simulink library "Kitchen_Lib"  (R2023a)
settings: Solver=VariableStepAuto  StartTime=0.0  StopTime=10.0  RelTol=1e-3  EnableMultiTasking=on
undefined symbols (not defined in the file): Kitc_BusTyp_P, Kitc_BusTypSkyr_C, Kitc_ColrLedColrls_C, Kitc_ColrLedGrn_C, Kitc_ColrLedRed_C, Kitc_ColrLedYlw_C, Kitc_StDgnWtrTank_C, Kitc_StElecPlugScktOffByClmp50_P, Kitc_StsDlyBlink_C, Kitc_StsErrBlink_C, Kitc_StsFctAcvn_P, Kitc_StsInfoBlink_C, Kitc_StsKitchnOffAutoIgOff_P, Kitc_StsKitchnOffBySwt_P, Kitc_StsKitchnOffDoorLockd_P, Kitc_StsKitchnOffIgOff_P, Kitc_StsKitchnOffUv_P, Kitc_StsKitchnOnBySwt_P, Kitc_StsKitchnOnNVM_P, Kitc_StsLedOff_C, Kitc_StsLedOn_C, Kitc_StsLrgCnsAcv_P, Kitc_StTrfrAnSwtInstd_P, Kitc_StTrfrSwtInstd_P, Kitc_TiKitcRefgtrOffDly_P, Kitc_ULowrThdBat_C, Kitc_UUpprThdBat_C, Kitc_ValFalse_C, Kitc_ValPwmFreq2_C, Kitc_ValPwmFreq_C, Kitc_ValTrue_C
libraries: MAN_Library x50, E2E_Lib x3
(part 9 of 13)

== system Kitchen_Lib/Kitchen/100ms/Kitchn/Subsystem1/Subsystem19/WaterTankEmptyDiagnostic/TurnOffDelay/TurnOffDelayOriginal ==
  TurnOffDelayEnable : Inport
  TurnOffDelayThreshold : Inport  Port=2
  CycleTime : Inport  Port=3
  Data Type Conversion1 : DataTypeConversion  OutDataTypeStr=uint32  SaturateOnIntegerOverflow=off  RndMeth=Floor
  Data Type Conversion2 : DataTypeConversion  OutDataTypeStr=boolean  SaturateOnIntegerOverflow=off  RndMeth=Floor
  Data Type Conversion3 : DataTypeConversion  OutDataTypeStr=uint32  SaturateOnIntegerOverflow=off  RndMeth=Floor
  FallingEdgeDetection : Subsystem  AncestorBlock=MAN_Library/FallingEdgeDetection
  Logical Operator2 : Logic  Operator=OR  AllPortsSameDT=off  OutDataTypeStr=boolean
  TimePulseOriginal : Subsystem  AncestorBlock=MAN_Library/BasicLibrary/TimePulseOriginal
  TurnOffDelayFlag : Outport
  TurnOffDelayExpiredTime : Outport  Port=2
  wires:
  CycleTime/1 -> TimePulseOriginal/3(CycleTime)
  Data Type Conversion3/1 -> TurnOffDelayExpiredTime/1
  Data Type Conversion1/1 -> TimePulseOriginal/2(TimePulseDuration)
  TurnOffDelayThreshold/1 -> Data Type Conversion1/1
  FallingEdgeDetection/1(Q) -> TimePulseOriginal/1(TimePulseEnable)
  TimePulseOriginal/2(TimePulseExpiredTime) -> Data Type Conversion3/1
  Logical Operator2/1 -> TurnOffDelayFlag/1
  TimePulseOriginal/1(TimePulseFlag) -> Logical Operator2/2
  Data Type Conversion2/1 -> FallingEdgeDetection/1(CLK), Logical Operator2/1
  TurnOffDelayEnable/1 -> Data Type Conversion2/1

== system Kitchen_Lib/Kitchen/100ms/Kitchn/Subsystem1/Subsystem16/001_KitchnCtl/002_FlipFlop/KSW-KitchenControl/KSW_Battery ==
  Kitchn_On : Inport
  "GW_Ubat " : Inport  Port=2
  GW_StClmp15 : Inport  Port=3
  "GW_StUvTopPrio " : Inport  Port=4
  "GW_ModeExbn " : Inport  Port=5
  "GW_StClmp50Off3Sec " : Inport  Port=6
  CLS_StDoorLockdOutd : Inport  Port=7
  Kitc_StsHostsCallAcv : Inport  Port=8
  GW_StEngRung : Inport  Port=9
  ABat_StAddlBatInstd : Inport  Port=10
  BatteryVoltageUnder22.7V : Subsystem
  BatteryVoltageUnder23V : Subsystem
  KitchenActivation : Subsystem
  Logical Operator51 : Logic  Operator=OR  AllPortsSameDT=off  OutDataTypeStr=boolean
  KitchnAcv : Outport
  LrgCnsEna : Outport  Port=2
  LrgCns : Outport  Port=3
  Kitc_WarnLrgCns : Outport  Port=4
  Kitc_StBuzRe : Outport  Port=5
  wires:
  Logical Operator51/1 -> BatteryVoltageUnder23V/2(EngOrAddlBat), KitchenActivation/9(EngOrAddlBat), BatteryVoltageUnder22.7V/2(EngOrAddlBat)
  "GW_Ubat "/1 -> BatteryVoltageUnder23V/1(GW_Ubat), BatteryVoltageUnder22.7V/3("GW_Ubat ")
  BatteryVoltageUnder22.7V/1(BatUUnder22.7V) -> KitchenActivation/5(BatUUnder22.7V)
  BatteryVoltageUnder23V/2(Kitc_WarnLrgCns) -> Kitc_WarnLrgCns/1
  BatteryVoltageUnder23V/3(Kitc_StBuzRe) -> Kitc_StBuzRe/1
  BatteryVoltageUnder23V/1(LrgCnsOff) -> KitchenActivation/6(LrgCnsOff)
  Kitchn_On/1 -> BatteryVoltageUnder22.7V/1(Kitchn_On), [Kitchn_On]
  [Kitchn_On] -> BatteryVoltageUnder23V/3(Kitchn_On)
  Kitc_StsHostsCallAcv/1 -> BatteryVoltageUnder23V/4(Kitc_StsHostsCallAcv)
  "GW_StClmp50Off3Sec "/1 -> KitchenActivation/1("GW_StClmp50Off3Sec ")
  "GW_StUvTopPrio "/1 -> KitchenActivation/2("GW_StUvTopPrio ")
  "GW_ModeExbn "/1 -> KitchenActivation/3("GW_ModeExbn ")
  CLS_StDoorLockdOutd/1 -> KitchenActivation/4(CLS_StDoorLockdOutd)
  GW_StClmp15/1 -> KitchenActivation/8(GW_StClmp15)
  KitchenActivation/1(KitchnAcv) -> KitchnAcv/1
  KitchenActivation/2(LrgCnsEna) -> LrgCnsEna/1
  KitchenActivation/3(LrgCns) -> LrgCns/1
  [Kitchn_On] -> KitchenActivation/7(Kitchn_On)
  ABat_StAddlBatInstd/1 -> Logical Operator51/1
  GW_StEngRung/1 -> Logical Operator51/2

== system Kitchen_Lib/Kitchen/100ms/Kitchn/Subsystem1/Subsystem16/001_KitchnCtl/002_FlipFlop/KSW-KitchenControl/KitchenControl ==
  Kitchn_On : Inport
  KitchnAcv : Inport  Port=2
  LrgCnsEna : Inport  Port=3
  "GW_ModeExbn " : Inport  Port=4
  GW_StClmp15 : Inport  Port=5
  ABat_StAddlBatInstd : Inport  Port=6
  GW_StEngRung : Inport  Port=7
  Constant : Constant  Value=Kitc_BusTypSkyr_C
  Constant1 : Constant  Value=Kitc_BusTypSkyr_C
  Constant2 : Constant  Value=Kitc_BusTyp_P
  Constant3 : Constant  Value=Kitc_BusTyp_P
  Constant4 : Constant  Value=Kitc_ValPwmFreq_C
  Gain : Gain  Gain=100  OutDataTypeStr=uint16
  Gain1 : Gain  Gain=100  OutDataTypeStr=uint16
  Logical Operator5 : Logic  Operator=OR  AllPortsSameDT=off  OutDataTypeStr=boolean
  Logical Operator50 : Logic  Inputs=3  AllPortsSameDT=off  OutDataTypeStr=boolean
  Logical Operator51 : Logic  Operator=OR  AllPortsSameDT=off  OutDataTypeStr=boolean
  Multiport Switch : MultiPortSwitch  DataPortOrder=Zero-based contiguous  Inputs=2  zeroidx=on  SaturateOnIntegerOverflow=off  InputSameDT=off
  Multiport Switch1 : MultiPortSwitch  DataPortOrder=Zero-based contiguous  Inputs=2  zeroidx=on  SaturateOnIntegerOverflow=off  InputSameDT=off
  Relational Operator : RelationalOperator  Operator===  OutDataTypeStr=boolean  InputSameDT=off
  Relational Operator1 : RelationalOperator  Operator===  OutDataTypeStr=boolean  InputSameDT=off
  Kitc_StsKitcAcv : Outport
  Kitchn_HostsCallOn : Outport  Port=2
  Kitc_StLrgCns : Outport  Port=3
  Kitc_StSmlCns : Outport  Port=4
  Kitc_StWtrPump : Outport  Port=5
  Kitc_StKitcLi : Outport  Port=6
  Kitc_StsPwmFreq : Outport  Port=7
  wires:
  Multiport Switch/1 -> Kitchn_HostsCallOn/1, Kitc_StsKitcAcv/1
  GW_StClmp15/1 -> Logical Operator50/1
  Constant/1 -> Relational Operator/2
  Logical Operator50/1 -> [SkylinerKitchnAcv]
  Multiport Switch1/1 -> Gain/1
  "GW_ModeExbn "/1 -> Logical Operator5/1
  Relational Operator1/1 -> Multiport Switch1/1
  Logical Operator5/1 -> Kitc_StKitcLi/1
  KitchnAcv/1 -> Logical Operator5/2, Gain1/1, Kitc_StWtrPump/1, Multiport Switch/2
  Kitchn_On/1 -> Logical Operator50/2
  Constant2/1 -> Relational Operator/1
  Logical Operator51/1 -> Logical Operator50/3
  Constant1/1 -> Relational Operator1/2
  Constant3/1 -> Relational Operator1/1
  Relational Operator/1 -> Multiport Switch/1
  [SkylinerKitchnAcv] -> Multiport Switch1/3
  [SkylinerKitchnAcv] -> Multiport Switch/3
  ABat_StAddlBatInstd/1 -> Logical Operator51/1
  GW_StEngRung/1 -> Logical Operator51/2
  LrgCnsEna/1 -> Multiport Switch1/2
  Gain/1 -> Kitc_StLrgCns/1
  Gain1/1 -> Kitc_StSmlCns/1
  Constant4/1 -> Kitc_StsPwmFreq/1

== system Kitchen_Lib/Kitchen/100ms/Kitchn/Subsystem1/Subsystem16/001_KitchnCtl/002_FlipFlop/KitchenEnable/KitchenOffAutomaticIgnitionOff ==
  Kitc_StDemoBd : Inport
  Kitc_TdOff : Inport  Port=2
  GW_StClmp15 : Inport  Port=3
  Kitchen_On : Inport  Port=4
  "Constant4           " : MAN_Library/TimeConstant  hours=0  minutes=0  seconds=10  miliseconds=0
  Logical Operator36 : Logic  AllPortsSameDT=off  OutDataTypeStr=boolean
  Logical Operator37 : Logic  Operator=NOT  Inputs=4  AllPortsSameDT=off  OutDataTypeStr=boolean
  Multiport Switch2 : MultiPortSwitch  DataPortOrder=Zero-based contiguous  Inputs=2  zeroidx=on  SaturateOnIntegerOverflow=off  InputSameDT=off
  RisingEdgeDetection2 : MAN_Library/RisingEdgeDetection
  Terminator : Terminator
  TurnOnDelay : MAN_Library/TurnOnDelay  CycleTime=Cycle Time: 10 Ms
  "KitchnOffAutoIgOff " : Outport
  wires:
  TurnOnDelay/1 -> RisingEdgeDetection2/1
  RisingEdgeDetection2/1 -> "KitchnOffAutoIgOff "/1
  Multiport Switch2/1 -> TurnOnDelay/2
  Logical Operator36/1 -> TurnOnDelay/1
  Logical Operator37/1 -> Logical Operator36/2
  TurnOnDelay/2 -> Terminator/1
  "Constant4           "/1 -> Multiport Switch2/3
  Kitc_StDemoBd/1 -> Multiport Switch2/1
  Kitc_TdOff/1 -> Multiport Switch2/2
  Kitchen_On/1 -> Logical Operator36/1
  GW_StClmp15/1 -> Logical Operator37/1

== system Kitchen_Lib/Kitchen/100ms/Kitchn/Subsystem1/Subsystem16/001_KitchnCtl/002_FlipFlop/KitchenEnable/KitchenOffBySwitch ==
  Kitc_StKitcSwtBotmPart : Inport
  "GW_ModeExbn " : Inport  Port=2
  Kitchen_On : Inport  Port=3
  Logical Operator20 : Logic  Inputs=3  AllPortsSameDT=off  OutDataTypeStr=boolean
  Logical Operator22 : Logic  Operator=NOT  Inputs=4  AllPortsSameDT=off  OutDataTypeStr=boolean
  RisingEdgeDetection : MAN_Library/RisingEdgeDetection
  KitchnOffBySwt : Outport
  wires:
  RisingEdgeDetection/1 -> Logical Operator20/1
  Logical Operator20/1 -> KitchnOffBySwt/1
  Logical Operator22/1 -> Logical Operator20/2
  "GW_ModeExbn "/1 -> Logical Operator22/1
  Kitc_StKitcSwtBotmPart/1 -> RisingEdgeDetection/1
  Kitchen_On/1 -> Logical Operator20/3

== system Kitchen_Lib/Kitchen/100ms/Kitchn/Subsystem1/Subsystem16/001_KitchnCtl/002_FlipFlop/KitchenEnable/KitchenOffDoorLocked ==
  CLS_StDoorLockdOutd : Inport
  GW_StClmp15 : Inport  Port=2
  Kitchen_On : Inport  Port=3
  Logical Operator39 : Logic  Inputs=3  AllPortsSameDT=off  OutDataTypeStr=boolean
  Logical Operator40 : Logic  Operator=NOT  Inputs=4  AllPortsSameDT=off  OutDataTypeStr=boolean
  RisingEdgeDetection3 : MAN_Library/RisingEdgeDetection
  KitchnOffDoorLockd : Outport
  wires:
  GW_StClmp15/1 -> Logical Operator40/1
  Kitchen_On/1 -> Logical Operator39/3
  Logical Operator39/1 -> KitchnOffDoorLockd/1
  RisingEdgeDetection3/1 -> Logical Operator39/2
  CLS_StDoorLockdOutd/1 -> RisingEdgeDetection3/1
  Logical Operator40/1 -> Logical Operator39/1

== system Kitchen_Lib/Kitchen/100ms/Kitchn/Subsystem1/Subsystem16/001_KitchnCtl/002_FlipFlop/KitchenEnable/KitchenOffIgnitionOff ==
  GW_StClmp15 : Inport
  Kitchen_On : Inport  Port=2
  FallingEdgeDetection : MAN_Library/FallingEdgeDetection
  Logical Operator31 : Logic  AllPortsSameDT=off  OutDataTypeStr=boolean
  KitchnOffIgOff : Outport
  wires:
  Kitchen_On/1 -> Logical Operator31/2
  FallingEdgeDetection/1 -> Logical Operator31/1
  Logical Operator31/1 -> KitchnOffIgOff/1
  GW_StClmp15/1 -> FallingEdgeDetection/1

== system Kitchen_Lib/Kitchen/100ms/Kitchn/Subsystem1/Subsystem16/001_KitchnCtl/002_FlipFlop/KitchenEnable/KitchenOffUndervoltage ==
  "GW_StUvTopPrio " : Inport
  Kitchen_On : Inport  Port=2
  Logical Operator38 : Logic  AllPortsSameDT=off  OutDataTypeStr=boolean
  RisingEdgeDetection4 : MAN_Library/RisingEdgeDetection
  KitchnOffUv : Outport
  wires:
  Logical Operator38/1 -> KitchnOffUv/1
  "GW_StUvTopPrio "/1 -> RisingEdgeDetection4/1
  RisingEdgeDetection4/1 -> Logical Operator38/2
  Kitchen_On/1 -> Logical Operator38/1

== system Kitchen_Lib/Kitchen/100ms/Kitchn/Subsystem1/Subsystem16/001_KitchnCtl/002_FlipFlop/KitchenEnable/KitchenOnBySwitch ==
  Kitc_StKitcSwtUpprPart : Inport
  "GW_ModeExbn " : Inport  Port=2
  "GW_StUvTopPrio " : Inport  Port=3
  Kitchn_On : Inport  Port=4
  Logical Operator : Logic  Inputs=4  AllPortsSameDT=off  OutDataTypeStr=boolean
  Logical Operator1 : Logic  Operator=NOT  Inputs=4  AllPortsSameDT=off  OutDataTypeStr=boolean
  Logical Operator2 : Logic  Operator=NOT  Inputs=4  AllPortsSameDT=off  OutDataTypeStr=boolean
  Logical Operator3 : Logic  Operator=NOT  Inputs=4  AllPortsSameDT=off  OutDataTypeStr=boolean
  RisingEdgeDetection : MAN_Library/RisingEdgeDetection
  "KitchnOnBySwt " : Outport
  wires:
  "GW_StUvTopPrio "/1 -> Logical Operator2/1
  Logical Operator/1 -> "KitchnOnBySwt "/1
  "GW_ModeExbn "/1 -> Logical Operator1/1
  Logical Operator2/1 -> Logical Operator/3
  Logical Operator3/1 -> Logical Operator/4
  Logical Operator1/1 -> Logical Operator/2
  Kitchn_On/1 -> Logical Operator3/1
  Kitc_StKitcSwtUpprPart/1 -> RisingEdgeDetection/1
  RisingEdgeDetection/1 -> Logical Operator/1

== system Kitchen_Lib/Kitchen/100ms/Kitchn/Subsystem1/Subsystem16/001_KitchnCtl/002_FlipFlop/KitchenEnable/KitchenOnNVM ==
  "GW_StStrtNew " : Inport
  "GW_ModeExbn " : Inport  Port=2
  GW_StClmp15 : Inport  Port=3
  Kitchen_On : Inport  Port=4
  KitchnOffBySwt : Inport  Port=5
  HostsSideBotmBtn_OFF : Inport  Port=6
  Kitc_ModeKitcNv : DataStoreWrite  DataStoreName=Kitc_ModeKitcNv  IndexOptions=Index vector (dialog)  Indices=1  OutputSizes=1
  Kitc_ModeKitcNv1 : DataStoreRead  DataStoreName=Kitc_ModeKitcNv  IndexOptions=Index vector (dialog)  Indices=1  OutputSizes=1
  Logical Operator32 : Logic  Inputs=5  AllPortsSameDT=off  OutDataTypeStr=boolean
  Logical Operator33 : Logic  Operator=NOT  Inputs=4  AllPortsSameDT=off  OutDataTypeStr=boolean
  Logical Operator34 : Logic  Operator=NOT  Inputs=4  AllPortsSameDT=off  OutDataTypeStr=boolean
  Logical Operator35 : Logic  Operator=NOT  Inputs=4  AllPortsSameDT=off  OutDataTypeStr=boolean
  NVM : Subsystem
  NvM_ActiveOnlyForFirstCycle : MAN_Library/NvM_ActiveOnlyForFirstCycle
  RisingEdgeDetection5 : MAN_Library/RisingEdgeDetection
  "KitchnOnNVM  " : Outport
  wires:
  "GW_ModeExbn "/1 -> Logical Operator34/1
  Logical Operator33/1 -> Logical Operator32/2
  RisingEdgeDetection5/1 -> Logical Operator32/1
  Logical Operator35/1 -> Logical Operator32/5
  "GW_StStrtNew "/1 -> NVM/3("GW_StStrtNew "), Logical Operator35/1
  Logical Operator34/1 -> Logical Operator32/3
  Logical Operator32/1 -> Kitc_ModeKitcNv/1, "KitchnOnNVM  "/1
  Kitchen_On/1 -> Logical Operator33/1, NVM/5(Kitchn_On)
  Kitc_ModeKitcNv1/1 -> NvM_ActiveOnlyForFirstCycle/1
  GW_StClmp15/1 -> RisingEdgeDetection5/1, NVM/6(GW_StClmp15)
  KitchnOffBySwt/1 -> NVM/1(KitchnOffBySwt)
  HostsSideBotmBtn_OFF/1 -> NVM/2(HostsSideBotmBtn_OFF)
  NvM_ActiveOnlyForFirstCycle/1 -> NVM/4(Kitc_ModeKitcNv), Logical Operator32/4

== system Kitchen_Lib/Kitchen/100ms/Kitchn/Subsystem1/Subsystem16/001_KitchnCtl/002_FlipFlop/KitchenEnable/Subsystem ==
  StateChange : Inport
  Ground : Ground
  Logical Operator : Logic  AllPortsSameDT=off  OutDataTypeStr=boolean
  RS : Subsystem  AncestorBlock=MAN_Library/RS
  RisingEdgeDetection : Subsystem  AncestorBlock=MAN_Library/RisingEdgeDetection
  StateChangePulse : Subsystem  AncestorBlock=MAN_Library/StateChangePulse
  Terminator : Terminator
  Terminator1 : Terminator
  TimeConstant : Subsystem  AncestorBlock=MAN_Library/TimeConstant  mask{hours=0, minutes=0, seconds=0, miliseconds=0}
      mask prompts: hours "Hour"
      mask DialogControl TimeConstant Prompt: Time Constant
      mask Display:
      | timeDraw = 'Time#';
      | if( hours == 0 && minutes == 0 && seconds == 0 && miliseconds == 0)
      |     timeDraw = strcat(timeDraw,'0secs'),
      | else
      |     if( hours ~= 0)
      |         timeDraw = strcat(timeDraw,num2str(hours),'hours');
      |     end
      |     if( minutes ~= 0)
      |         timeDraw = strcat(timeDraw,num2str(minutes),'min');
      |     end
      |     if( seconds ~= 0)
      |         timeDraw = strcat(timeDraw,num2str(seconds),'sec');
      |     end
      |     if( miliseconds ~= 0)
      |         timeDraw = strcat(timeDraw,num2str(miliseconds),'ms');
      |     end
      | end
      | fprintf(timeDraw);
  TurnOnDelay : Subsystem  AncestorBlock=MAN_Library/TurnOnDelay  mask(Turn On Delay){CycleTime=Cycle Time: 10 Ms}
      mask prompts: CycleTime "Select the Cycle Time:"
      mask help:
      | This is an EDGE DELAY where the turning-on edge is delayed. The delay period is entered at input PT. Output Q is set on TRUE after turning on input IN, only after the delay period is over. Output ET counts the time - beginning with the occurrence of the positive edge - until the value set at PT has been reached. The output ET shows the expired time since turning input IN on until the input state of IN is put through to output Q.
      |
      | IN : Timer starting bit
      | PT : Preset time of timer
      | Q  : Time up flag
      | ET : Current value of timer
      mask TypeOptions CycleTime: Cycle Time: 1 Ms | Cycle Time: 10 Ms | Cycle Time: 100 Ms | Cycle Time: 1000 Ms
      mask Display:
      | disp('{\bf\fontsize{18}Turn On Delay}', 'texmode','on');
      | 
      | port_label('input', 1,'IN');
      | port_label('input', 2,'PT');
      | port_label('output',1,'Q');
      | port_label('output',2,'ET');
  Unit Delay : UnitDelay  SampleTime=-1  HasFrameUpgradeWarning=on
  Kitchn_On : Outport
  wires:
  RS/1(Q) -> TurnOnDelay/1(TurnOnDelayEnable), Kitchn_On/1
  TimeConstant/1(time) -> TurnOnDelay/2(TurnOnDelayThreshold)
  TurnOnDelay/2(TurnOnDelayExpiredTime) -> Terminator/1
  TurnOnDelay/1(TurnOnDelayFlag) -> Unit Delay/1
  Unit Delay/1 -> Logical Operator/2
  Logical Operator/1 -> RS/2(R)
  RisingEdgeDetection/1(Q) -> Logical Operator/1, RS/1(S)
  StateChange/1 -> RisingEdgeDetection/1(CLK)
  Ground/1 -> StateChangePulse/1(IN)
  StateChangePulse/1(OUT) -> Terminator1/1

== system Kitchen_Lib/Kitchen/100ms/Kitchn/Subsystem1/Subsystem16/001_KitchnCtl/003_KitchenDriver/Diagnostic/DIAG ==
  In1 : Inport
  In2 : Inport  Port=2
  Dem_SetEventStatus : MAN_Library/Dem_SetEventStatus  Commented=on  SLB_DEMEventID=Kitc_StDgnWtrTank_C
  Terminator : Terminator
  Terminator1 : Terminator
  wires:
  In1/1 -> Terminator/1
  In2/1 -> Terminator1/1

== system Kitchen_Lib/Kitchen/100ms/Kitchn/Subsystem1/Subsystem19/KSW_Battery/BatteryVoltageUnder23V/TimePulse/TimePulseOriginal ==
  TimePulseEnable : Inport
  TimePulseDuration : Inport  Port=2
  CycleTime : Inport  Port=3
  Data Type Conversion1 : DataTypeConversion  OutDataTypeStr=uint32  SaturateOnIntegerOverflow=off  RndMeth=Floor
  Data Type Conversion2 : DataTypeConversion  OutDataTypeStr=boolean  SaturateOnIntegerOverflow=off  RndMeth=Floor
  Delay1 : Delay  DelayLength=1  InitialCondition=0  ExternalReset=Rising
      settings: InputPortMap=u0,r5
  Logical Operator1 : Logic  Operator=NOT  AllPortsSameDT=off  OutDataTypeStr=boolean
  Logical Operator2 : Logic  AllPortsSameDT=off  OutDataTypeStr=boolean
  RisingEdgeDetection : Subsystem  AncestorBlock=MAN_Library/RisingEdgeDetection
  RisingEdgeDetection1 : Subsystem  AncestorBlock=MAN_Library/RisingEdgeDetection
  SR : Subsystem  AncestorBlock=MAN_Library/SR
  TimerCountingUpOriginal : Subsystem  AncestorBlock=MAN_Library/BasicLibrary/TimerCountingUpOriginal
  TimePulseFlag : Outport
  TimePulseExpiredTime : Outport  Port=2
  wires:
  CycleTime/1 -> TimerCountingUpOriginal/4(CycleTime)
  Delay1/1 -> SR/2(R)
  [TimePulseReset] -> TimerCountingUpOriginal/2(TimerReset)
  [TimePulseReset] -> Delay1/2
  RisingEdgeDetection/1(Q) -> SR/1(S), [TimePulseReset]
  Data Type Conversion1/1 -> TimerCountingUpOriginal/3(TimerThreshold)
  Data Type Conversion2/1 -> RisingEdgeDetection/1(CLK)
  Logical Operator1/1 -> Logical Operator2/2
  Logical Operator2/1 -> TimePulseFlag/1
  RisingEdgeDetection1/1(Q) -> Delay1/1
  TimerCountingUpOriginal/1(TimerFlag) -> RisingEdgeDetection1/1(CLK), Logical Operator1/1
  SR/1(Q) -> Logical Operator2/1, TimerCountingUpOriginal/1(TimerEnable)
  TimePulseEnable/1 -> Data Type Conversion2/1
  TimePulseDuration/1 -> Data Type Conversion1/1
  TimerCountingUpOriginal/2(TimerCurrentValue) -> TimePulseExpiredTime/1

== system Kitchen_Lib/Kitchen/100ms/Kitchn/Subsystem1/Subsystem19/KSW_Battery/BatteryVoltageUnder23V/TimePulse1/TimePulseOriginal ==
  TimePulseEnable : Inport
  TimePulseDuration : Inport  Port=2
  CycleTime : Inport  Port=3
  Data Type Conversion1 : DataTypeConversion  OutDataTypeStr=uint32  SaturateOnIntegerOverflow=off  RndMeth=Floor
  Data Type Conversion2 : DataTypeConversion  OutDataTypeStr=boolean  SaturateOnIntegerOverflow=off  RndMeth=Floor
  Delay1 : Delay  DelayLength=1  InitialCondition=0  ExternalReset=Rising
      settings: InputPortMap=u0,r5
  Logical Operator1 : Logic  Operator=NOT  AllPortsSameDT=off  OutDataTypeStr=boolean
  Logical Operator2 : Logic  AllPortsSameDT=off  OutDataTypeStr=boolean
  RisingEdgeDetection : Subsystem  AncestorBlock=MAN_Library/RisingEdgeDetection
  RisingEdgeDetection1 : Subsystem  AncestorBlock=MAN_Library/RisingEdgeDetection
  SR : Subsystem  AncestorBlock=MAN_Library/SR
  TimerCountingUpOriginal : Subsystem  AncestorBlock=MAN_Library/BasicLibrary/TimerCountingUpOriginal
  TimePulseFlag : Outport
  TimePulseExpiredTime : Outport  Port=2
  wires:
  CycleTime/1 -> TimerCountingUpOriginal/4(CycleTime)
  Delay1/1 -> SR/2(R)
  [TimePulseReset] -> TimerCountingUpOriginal/2(TimerReset)
  [TimePulseReset] -> Delay1/2
  RisingEdgeDetection/1(Q) -> SR/1(S), [TimePulseReset]
  Data Type Conversion1/1 -> TimerCountingUpOriginal/3(TimerThreshold)
  Data Type Conversion2/1 -> RisingEdgeDetection/1(CLK)
  Logical Operator1/1 -> Logical Operator2/2
  Logical Operator2/1 -> TimePulseFlag/1
  RisingEdgeDetection1/1(Q) -> Delay1/1
  TimerCountingUpOriginal/1(TimerFlag) -> RisingEdgeDetection1/1(CLK), Logical Operator1/1
  SR/1(Q) -> Logical Operator2/1, TimerCountingUpOriginal/1(TimerEnable)
  TimePulseEnable/1 -> Data Type Conversion2/1
  TimePulseDuration/1 -> Data Type Conversion1/1
  TimerCountingUpOriginal/2(TimerCurrentValue) -> TimePulseExpiredTime/1

== system Kitchen_Lib/Kitchen/100ms/Kitchn/Subsystem1/Subsystem19/KSW_Battery/BatteryVoltageUnder23V/TurnOffDelay/TurnOffDelayOriginal ==
  TurnOffDelayEnable : Inport
  TurnOffDelayThreshold : Inport  Port=2
  CycleTime : Inport  Port=3
  Data Type Conversion1 : DataTypeConversion  OutDataTypeStr=uint32  SaturateOnIntegerOverflow=off  RndMeth=Floor
  Data Type Conversion2 : DataTypeConversion  OutDataTypeStr=boolean  SaturateOnIntegerOverflow=off  RndMeth=Floor
  Data Type Conversion3 : DataTypeConversion  OutDataTypeStr=uint32  SaturateOnIntegerOverflow=off  RndMeth=Floor
  FallingEdgeDetection : Subsystem  AncestorBlock=MAN_Library/FallingEdgeDetection
  Logical Operator2 : Logic  Operator=OR  AllPortsSameDT=off  OutDataTypeStr=boolean
  TimePulseOriginal : Subsystem  AncestorBlock=MAN_Library/BasicLibrary/TimePulseOriginal
  TurnOffDelayFlag : Outport
  TurnOffDelayExpiredTime : Outport  Port=2
  wires:
  CycleTime/1 -> TimePulseOriginal/3(CycleTime)
  Data Type Conversion3/1 -> TurnOffDelayExpiredTime/1
  Data Type Conversion1/1 -> TimePulseOriginal/2(TimePulseDuration)
  TurnOffDelayThreshold/1 -> Data Type Conversion1/1
  FallingEdgeDetection/1(Q) -> TimePulseOriginal/1(TimePulseEnable)
  TimePulseOriginal/2(TimePulseExpiredTime) -> Data Type Conversion3/1
  Logical Operator2/1 -> TurnOffDelayFlag/1
  TimePulseOriginal/1(TimePulseFlag) -> Logical Operator2/2
  Data Type Conversion2/1 -> FallingEdgeDetection/1(CLK), Logical Operator2/1
  TurnOffDelayEnable/1 -> Data Type Conversion2/1

== system Kitchen_Lib/Kitchen/100ms/Kitchn/Subsystem1/Subsystem19/KitchenEnable/001_HostessSideButton/001_HostessSideTopButton/RisingEdgeDetection ==
  CLK : Inport
  Constant : Constant  Value=boolean(1)  OutDataTypeStr=boolean
  Data Type Conversion1 : DataTypeConversion  OutDataTypeStr=boolean  SaturateOnIntegerOverflow=off  RndMeth=Floor
  Logical Operator : Logic  AllPortsSameDT=off  OutDataTypeStr=boolean
  Relational Operator : RelationalOperator  Operator=~=  OutDataTypeStr=boolean  InputSameDT=off
  Relational Operator1 : RelationalOperator  Operator===  OutDataTypeStr=boolean  InputSameDT=off
  Unit Delay : UnitDelay  SampleTime=-1  HasFrameUpgradeWarning=on
  Q : Outport
  wires:
  CLK/1 -> Data Type Conversion1/1
  Unit Delay/1 -> Relational Operator/1
  Relational Operator/1 -> Logical Operator/1
  Relational Operator1/1 -> Logical Operator/2
  Logical Operator/1 -> Q/1
  Constant/1 -> Relational Operator1/2
  Data Type Conversion1/1 -> Unit Delay/1, Relational Operator/2, Relational Operator1/1

== system Kitchen_Lib/Kitchen/100ms/Kitchn/Subsystem1/Subsystem19/KitchenEnable/001_HostessSideButton/002_HostessSideBottomButton/RisingEdgeDetection ==
  CLK : Inport
  Constant : Constant  Value=boolean(1)  OutDataTypeStr=boolean
  Data Type Conversion1 : DataTypeConversion  OutDataTypeStr=boolean  SaturateOnIntegerOverflow=off  RndMeth=Floor
  Logical Operator : Logic  AllPortsSameDT=off  OutDataTypeStr=boolean
  Relational Operator : RelationalOperator  Operator=~=  OutDataTypeStr=boolean  InputSameDT=off
  Relational Operator1 : RelationalOperator  Operator===  OutDataTypeStr=boolean  InputSameDT=off
  Unit Delay : UnitDelay  SampleTime=-1  HasFrameUpgradeWarning=on
  Q : Outport
  wires:
  CLK/1 -> Data Type Conversion1/1
  Unit Delay/1 -> Relational Operator/1
  Relational Operator/1 -> Logical Operator/1
  Relational Operator1/1 -> Logical Operator/2
  Logical Operator/1 -> Q/1
  Constant/1 -> Relational Operator1/2
  Data Type Conversion1/1 -> Unit Delay/1, Relational Operator/2, Relational Operator1/1

== system Kitchen_Lib/Kitchen/100ms/Kitchn/Subsystem1/Subsystem19/KitchenEnable/KitchenOffAutomaticIgnitionOff/TurnOnDelay/TurnOnDelayOriginal ==
  TurnOnDelayEnable : Inport
  TurnOnDelayThreshold : Inport  Port=2
  CycleTime : Inport  Port=3
  Data Type Conversion1 : DataTypeConversion  OutDataTypeStr=uint32  SaturateOnIntegerOverflow=off  RndMeth=Floor
  Data Type Conversion2 : DataTypeConversion  OutDataTypeStr=boolean  SaturateOnIntegerOverflow=off  RndMeth=Floor
  Logical Operator1 : Logic  Operator=NOT  AllPortsSameDT=off  OutDataTypeStr=boolean
  Logical Operator2 : Logic  AllPortsSameDT=off  OutDataTypeStr=boolean
  RisingEdgeDetection : Subsystem  AncestorBlock=MAN_Library/RisingEdgeDetection
  TimePulseOriginal : Subsystem  AncestorBlock=MAN_Library/BasicLibrary/TimePulseOriginal
  TurnOnDelayFlag : Outport
  TurnOnDelayExpiredTime : Outport  Port=2
  wires:
  CycleTime/1 -> TimePulseOriginal/3(CycleTime)
  Logical Operator2/1 -> TurnOnDelayFlag/1
  TimePulseOriginal/1(TimePulseFlag) -> Logical Operator1/1
  Logical Operator1/1 -> Logical Operator2/2
  TimePulseOriginal/2(TimePulseExpiredTime) -> TurnOnDelayExpiredTime/1
  RisingEdgeDetection/1(Q) -> TimePulseOriginal/1(TimePulseEnable)
  Data Type Conversion1/1 -> TimePulseOriginal/2(TimePulseDuration)
  TurnOnDelayThreshold/1 -> Data Type Conversion1/1
  TurnOnDelayEnable/1 -> Data Type Conversion2/1
  Data Type Conversion2/1 -> RisingEdgeDetection/1(CLK), Logical Operator2/1

== system Kitchen_Lib/Kitchen/100ms/Kitchn/Subsystem1/Subsystem19/KitchenEnable/KitchenOnNVM/NVM/RisingEdgeDetection1 ==
  CLK : Inport
  Constant : Constant  Value=boolean(1)  OutDataTypeStr=boolean
  Data Type Conversion1 : DataTypeConversion  OutDataTypeStr=boolean  SaturateOnIntegerOverflow=off  RndMeth=Floor
  Logical Operator : Logic  AllPortsSameDT=off  OutDataTypeStr=boolean
  Relational Operator : RelationalOperator  Operator=~=  OutDataTypeStr=boolean  InputSameDT=off
  Relational Operator1 : RelationalOperator  Operator===  OutDataTypeStr=boolean  InputSameDT=off
  Unit Delay : UnitDelay  SampleTime=-1  HasFrameUpgradeWarning=on
  Q : Outport
  wires:
  CLK/1 -> Data Type Conversion1/1
  Unit Delay/1 -> Relational Operator/1
  Relational Operator/1 -> Logical Operator/1
  Relational Operator1/1 -> Logical Operator/2
  Logical Operator/1 -> Q/1
  Constant/1 -> Relational Operator1/2
  Data Type Conversion1/1 -> Unit Delay/1, Relational Operator/2, Relational Operator1/1

== system Kitchen_Lib/Kitchen/100ms/Kitchn/Subsystem1/Subsystem19/KitchenEnable/KitchenOnNVM/NVM/RisingEdgeDetection2 ==
  CLK : Inport
  Constant : Constant  Value=boolean(1)  OutDataTypeStr=boolean
  Data Type Conversion1 : DataTypeConversion  OutDataTypeStr=boolean  SaturateOnIntegerOverflow=off  RndMeth=Floor
  Logical Operator : Logic  AllPortsSameDT=off  OutDataTypeStr=boolean
  Relational Operator : RelationalOperator  Operator=~=  OutDataTypeStr=boolean  InputSameDT=off
  Relational Operator1 : RelationalOperator  Operator===  OutDataTypeStr=boolean  InputSameDT=off
  Unit Delay : UnitDelay  SampleTime=-1  HasFrameUpgradeWarning=on
  Q : Outport
  wires:
  CLK/1 -> Data Type Conversion1/1
  Unit Delay/1 -> Relational Operator/1
  Relational Operator/1 -> Logical Operator/1
  Relational Operator1/1 -> Logical Operator/2
  Logical Operator/1 -> Q/1
  Constant/1 -> Relational Operator1/2
  Data Type Conversion1/1 -> Unit Delay/1, Relational Operator/2, Relational Operator1/1

== system Kitchen_Lib/Kitchen/100ms/Kitchn/Subsystem1/Subsystem19/KitchenEnable/KitchenOnNVM/NvM_ActiveOnlyForFirstCycle/Unit Delay External IC ==
  note: Initial Value
  note: Xnew
  u : Inport
  IC : Inport  Port=2
  FixPt Constant : Constant  DisableCoverage=on  Value=0  OutDataTypeStr=fixdt(0,8,0)
  FixPt Data Type Duplicate1 : DataTypeDuplicate  DisableCoverage=on  NumInputPorts=3
  FixPt Unit Delay1 : UnitDelay  DisableCoverage=on  InitialCondition=0.0  SampleTime=tsamp
  FixPt Unit Delay2 : UnitDelay  DisableCoverage=on  InitialCondition=1  SampleTime=tsamp  HasFrameUpgradeWarning=on
  Init : Switch  Criteria=u2 ~= 0  OutDataTypeStr=Inherit: Inherit via back propagation  ZeroCross=off  SaturateOnIntegerOverflow=off  InputSameDT=off
  y : Outport
  wires:
  IC/1 -> FixPt Data Type Duplicate1/3, Init/1
  u/1 -> FixPt Data Type Duplicate1/2, FixPt Unit Delay1/1
  FixPt Constant/1 -> FixPt Unit Delay2/1
  FixPt Unit Delay2/1 -> Init/2
  Init/1 -> FixPt Data Type Duplicate1/1, y/1
  FixPt Unit Delay1/1 -> Init/3  "Xold"

== system Kitchen_Lib/Kitchen/100ms/Kitchn/Subsystem1/Subsystem19/KitchenEnable/Subsystem/TurnOnDelay/TurnOnDelayOriginal ==
  TurnOnDelayEnable : Inport
  TurnOnDelayThreshold : Inport  Port=2
  CycleTime : Inport  Port=3
  Data Type Conversion1 : DataTypeConversion  OutDataTypeStr=uint32  SaturateOnIntegerOverflow=off  RndMeth=Floor
  Data Type Conversion2 : DataTypeConversion  OutDataTypeStr=boolean  SaturateOnIntegerOverflow=off  RndMeth=Floor
  Logical Operator1 : Logic  Operator=NOT  AllPortsSameDT=off  OutDataTypeStr=boolean
  Logical Operator2 : Logic  AllPortsSameDT=off  OutDataTypeStr=boolean
  RisingEdgeDetection : Subsystem  AncestorBlock=MAN_Library/RisingEdgeDetection
  TimePulseOriginal : Subsystem  AncestorBlock=MAN_Library/BasicLibrary/TimePulseOriginal
  TurnOnDelayFlag : Outport
  TurnOnDelayExpiredTime : Outport  Port=2
  wires:
  CycleTime/1 -> TimePulseOriginal/3(CycleTime)
  Logical Operator2/1 -> TurnOnDelayFlag/1
  TimePulseOriginal/1(TimePulseFlag) -> Logical Operator1/1
  Logical Operator1/1 -> Logical Operator2/2
  TimePulseOriginal/2(TimePulseExpiredTime) -> TurnOnDelayExpiredTime/1
  RisingEdgeDetection/1(Q) -> TimePulseOriginal/1(TimePulseEnable)
  Data Type Conversion1/1 -> TimePulseOriginal/2(TimePulseDuration)
  TurnOnDelayThreshold/1 -> Data Type Conversion1/1
  TurnOnDelayEnable/1 -> Data Type Conversion2/1
  Data Type Conversion2/1 -> RisingEdgeDetection/1(CLK), Logical Operator2/1

== system Kitchen_Lib/Kitchen/100ms/Kitchn/Subsystem1/Subsystem19/KitchenSwtLed/KitchenError/TurnOffDelay/TurnOffDelayOriginal ==
  TurnOffDelayEnable : Inport
  TurnOffDelayThreshold : Inport  Port=2
  CycleTime : Inport  Port=3
  Data Type Conversion1 : DataTypeConversion  OutDataTypeStr=uint32  SaturateOnIntegerOverflow=off  RndMeth=Floor
  Data Type Conversion2 : DataTypeConversion  OutDataTypeStr=boolean  SaturateOnIntegerOverflow=off  RndMeth=Floor
  Data Type Conversion3 : DataTypeConversion  OutDataTypeStr=uint32  SaturateOnIntegerOverflow=off  RndMeth=Floor
  FallingEdgeDetection : Subsystem  AncestorBlock=MAN_Library/FallingEdgeDetection
  Logical Operator2 : Logic  Operator=OR  AllPortsSameDT=off  OutDataTypeStr=boolean
  TimePulseOriginal : Subsystem  AncestorBlock=MAN_Library/BasicLibrary/TimePulseOriginal
  TurnOffDelayFlag : Outport
  TurnOffDelayExpiredTime : Outport  Port=2
  wires:
  CycleTime/1 -> TimePulseOriginal/3(CycleTime)
  Data Type Conversion3/1 -> TurnOffDelayExpiredTime/1
  Data Type Conversion1/1 -> TimePulseOriginal/2(TimePulseDuration)
  TurnOffDelayThreshold/1 -> Data Type Conversion1/1
  FallingEdgeDetection/1(Q) -> TimePulseOriginal/1(TimePulseEnable)
  TimePulseOriginal/2(TimePulseExpiredTime) -> Data Type Conversion3/1
  Logical Operator2/1 -> TurnOffDelayFlag/1
  TimePulseOriginal/1(TimePulseFlag) -> Logical Operator2/2
  Data Type Conversion2/1 -> FallingEdgeDetection/1(CLK), Logical Operator2/1
  TurnOffDelayEnable/1 -> Data Type Conversion2/1

== system Kitchen_Lib/Kitchen/100ms/Kitchn/Subsystem1/Subsystem19/KitchenSwtLed/TurnOffDelay1/TurnOffDelayOriginal/FallingEdgeDetection ==
  CLK : Inport
  Constant : Constant  Value=boolean(0)  OutDataTypeStr=boolean
  Data Type Conversion1 : DataTypeConversion  OutDataTypeStr=boolean  SaturateOnIntegerOverflow=off  RndMeth=Floor
  Logical Operator1 : Logic  AllPortsSameDT=off  OutDataTypeStr=boolean
  Relational Operator2 : RelationalOperator  Operator=~=  OutDataTypeStr=boolean  InputSameDT=off
  Relational Operator3 : RelationalOperator  Operator===  OutDataTypeStr=boolean  InputSameDT=off
  Unit Delay1 : UnitDelay  SampleTime=-1  HasFrameUpgradeWarning=on
  Q : Outport
  wires:
  Data Type Conversion1/1 -> Unit Delay1/1, Relational Operator2/2, Relational Operator3/1
  Constant/1 -> Relational Operator3/2
  CLK/1 -> Data Type Conversion1/1
  Logical Operator1/1 -> Q/1
  Relational Operator3/1 -> Logical Operator1/2
  Relational Operator2/1 -> Logical Operator1/1
  Unit Delay1/1 -> Relational Operator2/1

== system Kitchen_Lib/Kitchen/100ms/Kitchn/Subsystem1/Subsystem19/KitchenSwtLed/TurnOffDelay1/TurnOffDelayOriginal/TimePulseOriginal ==
  TimePulseEnable : Inport
  TimePulseDuration : Inport  Port=2
  CycleTime : Inport  Port=3
  Data Type Conversion1 : DataTypeConversion  OutDataTypeStr=uint32  SaturateOnIntegerOverflow=off  RndMeth=Floor
  Data Type Conversion2 : DataTypeConversion  OutDataTypeStr=boolean  SaturateOnIntegerOverflow=off  RndMeth=Floor
  Delay1 : Delay  DelayLength=1  InitialCondition=0  ExternalReset=Rising
      settings: InputPortMap=u0,r5
  Logical Operator1 : Logic  Operator=NOT  AllPortsSameDT=off  OutDataTypeStr=boolean
  Logical Operator2 : Logic  AllPortsSameDT=off  OutDataTypeStr=boolean
  RisingEdgeDetection : Subsystem  AncestorBlock=MAN_Library/RisingEdgeDetection
  RisingEdgeDetection1 : Subsystem  AncestorBlock=MAN_Library/RisingEdgeDetection
  SR : Subsystem  AncestorBlock=MAN_Library/SR
  TimerCountingUpOriginal : Subsystem  AncestorBlock=MAN_Library/BasicLibrary/TimerCountingUpOriginal
  TimePulseFlag : Outport
  TimePulseExpiredTime : Outport  Port=2
  wires:
  CycleTime/1 -> TimerCountingUpOriginal/4(CycleTime)
  Delay1/1 -> SR/2(R)
  [TimePulseReset] -> TimerCountingUpOriginal/2(TimerReset)
  [TimePulseReset] -> Delay1/2
  RisingEdgeDetection/1(Q) -> SR/1(S), [TimePulseReset]
  Data Type Conversion1/1 -> TimerCountingUpOriginal/3(TimerThreshold)
  Data Type Conversion2/1 -> RisingEdgeDetection/1(CLK)
  Logical Operator1/1 -> Logical Operator2/2
  Logical Operator2/1 -> TimePulseFlag/1
  RisingEdgeDetection1/1(Q) -> Delay1/1
  TimerCountingUpOriginal/1(TimerFlag) -> RisingEdgeDetection1/1(CLK), Logical Operator1/1
  SR/1(Q) -> Logical Operator2/1, TimerCountingUpOriginal/1(TimerEnable)
  TimePulseEnable/1 -> Data Type Conversion2/1
  TimePulseDuration/1 -> Data Type Conversion1/1
  TimerCountingUpOriginal/2(TimerCurrentValue) -> TimePulseExpiredTime/1

== system Kitchen_Lib/Kitchen/100ms/Kitchn/Subsystem1/Subsystem19/Refgtr/TurnOffDelay/TurnOffDelayOriginal/FallingEdgeDetection ==
  CLK : Inport
  Constant : Constant  Value=boolean(0)  OutDataTypeStr=boolean
  Data Type Conversion1 : DataTypeConversion  OutDataTypeStr=boolean  SaturateOnIntegerOverflow=off  RndMeth=Floor
  Logical Operator1 : Logic  AllPortsSameDT=off  OutDataTypeStr=boolean
  Relational Operator2 : RelationalOperator  Operator=~=  OutDataTypeStr=boolean  InputSameDT=off
  Relational Operator3 : RelationalOperator  Operator===  OutDataTypeStr=boolean  InputSameDT=off
  Unit Delay1 : UnitDelay  SampleTime=-1  HasFrameUpgradeWarning=on
  Q : Outport
  wires:
  Data Type Conversion1/1 -> Unit Delay1/1, Relational Operator2/2, Relational Operator3/1
  Constant/1 -> Relational Operator3/2
  CLK/1 -> Data Type Conversion1/1
  Logical Operator1/1 -> Q/1
  Relational Operator3/1 -> Logical Operator1/2
  Relational Operator2/1 -> Logical Operator1/1
  Unit Delay1/1 -> Relational Operator2/1

== system Kitchen_Lib/Kitchen/100ms/Kitchn/Subsystem1/Subsystem19/Refgtr/TurnOffDelay/TurnOffDelayOriginal/TimePulseOriginal ==
  TimePulseEnable : Inport
  TimePulseDuration : Inport  Port=2
  CycleTime : Inport  Port=3
  Data Type Conversion1 : DataTypeConversion  OutDataTypeStr=uint32  SaturateOnIntegerOverflow=off  RndMeth=Floor
  Data Type Conversion2 : DataTypeConversion  OutDataTypeStr=boolean  SaturateOnIntegerOverflow=off  RndMeth=Floor
  Delay1 : Delay  DelayLength=1  InitialCondition=0  ExternalReset=Rising
      settings: InputPortMap=u0,r5
  Logical Operator1 : Logic  Operator=NOT  AllPortsSameDT=off  OutDataTypeStr=boolean
  Logical Operator2 : Logic  AllPortsSameDT=off  OutDataTypeStr=boolean
  RisingEdgeDetection : Subsystem  AncestorBlock=MAN_Library/RisingEdgeDetection
  RisingEdgeDetection1 : Subsystem  AncestorBlock=MAN_Library/RisingEdgeDetection
  SR : Subsystem  AncestorBlock=MAN_Library/SR
  TimerCountingUpOriginal : Subsystem  AncestorBlock=MAN_Library/BasicLibrary/TimerCountingUpOriginal
  TimePulseFlag : Outport
  TimePulseExpiredTime : Outport  Port=2
  wires:
  CycleTime/1 -> TimerCountingUpOriginal/4(CycleTime)
  Delay1/1 -> SR/2(R)
  [TimePulseReset] -> TimerCountingUpOriginal/2(TimerReset)
  [TimePulseReset] -> Delay1/2
  RisingEdgeDetection/1(Q) -> SR/1(S), [TimePulseReset]
  Data Type Conversion1/1 -> TimerCountingUpOriginal/3(TimerThreshold)
  Data Type Conversion2/1 -> RisingEdgeDetection/1(CLK)
  Logical Operator1/1 -> Logical Operator2/2
  Logical Operator2/1 -> TimePulseFlag/1
  RisingEdgeDetection1/1(Q) -> Delay1/1
  TimerCountingUpOriginal/1(TimerFlag) -> RisingEdgeDetection1/1(CLK), Logical Operator1/1
  SR/1(Q) -> Logical Operator2/1, TimerCountingUpOriginal/1(TimerEnable)
  TimePulseEnable/1 -> Data Type Conversion2/1
  TimePulseDuration/1 -> Data Type Conversion1/1
  TimerCountingUpOriginal/2(TimerCurrentValue) -> TimePulseExpiredTime/1

== system Kitchen_Lib/Kitchen/100ms/Kitchn/Subsystem1/Subsystem19/TimePulse/TimePulseOriginal/TimerCountingUpOriginal/RisingEdgeDetection ==
  CLK : Inport
  Constant : Constant  Value=boolean(1)  OutDataTypeStr=boolean
  Data Type Conversion1 : DataTypeConversion  OutDataTypeStr=boolean  SaturateOnIntegerOverflow=off  RndMeth=Floor
  Logical Operator : Logic  AllPortsSameDT=off  OutDataTypeStr=boolean
  Relational Operator : RelationalOperator  Operator=~=  OutDataTypeStr=boolean  InputSameDT=off
  Relational Operator1 : RelationalOperator  Operator===  OutDataTypeStr=boolean  InputSameDT=off
  Unit Delay : UnitDelay  SampleTime=-1  HasFrameUpgradeWarning=on
  Q : Outport
  wires:
  Data Type Conversion1/1 -> Relational Operator1/1, Relational Operator/2, Unit Delay/1
  Constant/1 -> Relational Operator1/2
  Logical Operator/1 -> Q/1
  Relational Operator1/1 -> Logical Operator/2
  Relational Operator/1 -> Logical Operator/1
  Unit Delay/1 -> Relational Operator/1
  CLK/1 -> Data Type Conversion1/1

== system Kitchen_Lib/Kitchen/100ms/Kitchn/Subsystem1/Subsystem19/TimePulse/TimePulseOriginal/TimerCountingUpOriginal/U32_Saturation ==
  UpperLimit : Inport
  IN : Inport  Port=2
  LowerLimit : Inport  Port=3
  Data Type Conversion{1..4} (4 alike) : DataTypeConversion  OutDataTypeStr=uint32  SaturateOnIntegerOverflow=off  RndMeth=Floor
  MinMax : MinMax  Inputs=2  OutDataTypeStr=uint32
  MinMax1 : MinMax  Function=max  Inputs=2  OutDataTypeStr=uint32
  OUT : Outport
  wires:
  Data Type Conversion3/1 -> OUT/1
  Data Type Conversion2/1 -> MinMax/1
  Data Type Conversion1/1 -> MinMax/2
  Data Type Conversion4/1 -> MinMax1/1
  MinMax1/1 -> Data Type Conversion3/1
  LowerLimit/1 -> Data Type Conversion4/1
  MinMax/1 -> MinMax1/2
  IN/1 -> Data Type Conversion2/1
  UpperLimit/1 -> Data Type Conversion1/1

== system Kitchen_Lib/Kitchen/100ms/Kitchn/Subsystem1/Subsystem19/Trfr/002_FlipFlop/KSW-Nvm/SR ==
  S : Inport
  R : Inport  Port=2
  Constant1 : Constant  Value=boolean(1)  OutDataTypeStr=boolean
  Constant3 : Constant  Value=boolean(0)  OutDataTypeStr=boolean
  Data Type Conversion1 : DataTypeConversion  OutDataTypeStr=boolean  SaturateOnIntegerOverflow=off  RndMeth=Floor
  Data Type Conversion2 : DataTypeConversion  OutDataTypeStr=boolean  SaturateOnIntegerOverflow=off  RndMeth=Floor
  Multiport Switch : MultiPortSwitch  DataPortOrder=Zero-based contiguous  Inputs=2  zeroidx=on  SaturateOnIntegerOverflow=off  InputSameDT=off
  Multiport Switch1 : MultiPortSwitch  DataPortOrder=Zero-based contiguous  Inputs=2  zeroidx=on  SaturateOnIntegerOverflow=off  InputSameDT=off
  Unit Delay : UnitDelay  SampleTime=-1  HasFrameUpgradeWarning=on
  Q : Outport
  wires:
  S/1 -> Data Type Conversion2/1
  Constant1/1 -> Multiport Switch/3
  Multiport Switch1/1 -> Multiport Switch/2
  R/1 -> Data Type Conversion1/1
  Unit Delay/1 -> Multiport Switch1/2
  Multiport Switch/1 -> Q/1, Unit Delay/1
  Constant3/1 -> Multiport Switch1/3
  Data Type Conversion1/1 -> Multiport Switch1/1
  Data Type Conversion2/1 -> Multiport Switch/1

== system Kitchen_Lib/Kitchen/100ms/Kitchn/Subsystem1/Subsystem19/Trfr/002_FlipFlop/NvM_ActiveOnlyForFirstCycle/Unit Delay External IC ==
  note: Initial Value
  note: Xnew
  u : Inport
  IC : Inport  Port=2
  FixPt Constant : Constant  DisableCoverage=on  Value=0  OutDataTypeStr=fixdt(0,8,0)
  FixPt Data Type Duplicate1 : DataTypeDuplicate  DisableCoverage=on  NumInputPorts=3
  FixPt Unit Delay1 : UnitDelay  DisableCoverage=on  InitialCondition=0.0  SampleTime=tsamp
  FixPt Unit Delay2 : UnitDelay  DisableCoverage=on  InitialCondition=1  SampleTime=tsamp  HasFrameUpgradeWarning=on
  Init : Switch  Criteria=u2 ~= 0  OutDataTypeStr=Inherit: Inherit via back propagation  ZeroCross=off  SaturateOnIntegerOverflow=off  InputSameDT=off
  y : Outport
  wires:
  IC/1 -> FixPt Data Type Duplicate1/3, Init/1
  u/1 -> FixPt Data Type Duplicate1/2, FixPt Unit Delay1/1
  FixPt Constant/1 -> FixPt Unit Delay2/1
  FixPt Unit Delay2/1 -> Init/2
  Init/1 -> FixPt Data Type Duplicate1/1, y/1
  FixPt Unit Delay1/1 -> Init/3  "Xold"

== system Kitchen_Lib/Kitchen/100ms/Kitchn/Subsystem1/Subsystem19/Trfr/002_FlipFlop/TurnOffByButton/RisingEdgeDetection1 ==
  CLK : Inport
  Constant : Constant  Value=boolean(1)  OutDataTypeStr=boolean
  Data Type Conversion1 : DataTypeConversion  OutDataTypeStr=boolean  SaturateOnIntegerOverflow=off  RndMeth=Floor
  Logical Operator : Logic  AllPortsSameDT=off  OutDataTypeStr=boolean
  Relational Operator : RelationalOperator  Operator=~=  OutDataTypeStr=boolean  InputSameDT=off
  Relational Operator1 : RelationalOperator  Operator===  OutDataTypeStr=boolean  InputSameDT=off
  Unit Delay : UnitDelay  SampleTime=-1  HasFrameUpgradeWarning=on
  Q : Outport
  wires:
  CLK/1 -> Data Type Conversion1/1
  Unit Delay/1 -> Relational Operator/1
  Relational Operator/1 -> Logical Operator/1
  Relational Operator1/1 -> Logical Operator/2
  Logical Operator/1 -> Q/1
  Constant/1 -> Relational Operator1/2
  Data Type Conversion1/1 -> Unit Delay/1, Relational Operator/2, Relational Operator1/1

== system Kitchen_Lib/Kitchen/100ms/Kitchn/Subsystem1/Subsystem19/Trfr/002_FlipFlop/TurnOffConditions/FallingEdgeDetection ==
  CLK : Inport
  Constant : Constant  Value=boolean(0)  OutDataTypeStr=boolean
  Data Type Conversion1 : DataTypeConversion  OutDataTypeStr=boolean  SaturateOnIntegerOverflow=off  RndMeth=Floor
  Logical Operator1 : Logic  AllPortsSameDT=off  OutDataTypeStr=boolean
  Relational Operator2 : RelationalOperator  Operator=~=  OutDataTypeStr=boolean  InputSameDT=off
  Relational Operator3 : RelationalOperator  Operator===  OutDataTypeStr=boolean  InputSameDT=off
  Unit Delay1 : UnitDelay  SampleTime=-1  HasFrameUpgradeWarning=on
  Q : Outport
  wires:
  Unit Delay1/1 -> Relational Operator2/1
  Relational Operator2/1 -> Logical Operator1/1
  Relational Operator3/1 -> Logical Operator1/2
  Logical Operator1/1 -> Q/1
  CLK/1 -> Data Type Conversion1/1
  Constant/1 -> Relational Operator3/2
  Data Type Conversion1/1 -> Relational Operator3/1, Relational Operator2/2, Unit Delay1/1

== system Kitchen_Lib/Kitchen/100ms/Kitchn/Subsystem1/Subsystem19/Trfr/002_FlipFlop/TurnOffConditions/FallingEdgeDetection1 ==
  CLK : Inport
  Constant : Constant  Value=boolean(0)  OutDataTypeStr=boolean
  Data Type Conversion1 : DataTypeConversion  OutDataTypeStr=boolean  SaturateOnIntegerOverflow=off  RndMeth=Floor
  Logical Operator1 : Logic  AllPortsSameDT=off  OutDataTypeStr=boolean
  Relational Operator2 : RelationalOperator  Operator=~=  OutDataTypeStr=boolean  InputSameDT=off
  Relational Operator3 : RelationalOperator  Operator===  OutDataTypeStr=boolean  InputSameDT=off
  Unit Delay1 : UnitDelay  SampleTime=-1  HasFrameUpgradeWarning=on
  Q : Outport
  wires:
  Unit Delay1/1 -> Relational Operator2/1
  Relational Operator2/1 -> Logical Operator1/1
  Relational Operator3/1 -> Logical Operator1/2
  Logical Operator1/1 -> Q/1
  CLK/1 -> Data Type Conversion1/1
  Constant/1 -> Relational Operator3/2
  Data Type Conversion1/1 -> Relational Operator3/1, Relational Operator2/2, Unit Delay1/1

== system Kitchen_Lib/Kitchen/100ms/Kitchn/Subsystem1/Subsystem19/Trfr/002_FlipFlop/TurnOffConditions/RisingEdgeDetection2 ==
  CLK : Inport
  Constant : Constant  Value=boolean(1)  OutDataTypeStr=boolean
  Data Type Conversion1 : DataTypeConversion  OutDataTypeStr=boolean  SaturateOnIntegerOverflow=off  RndMeth=Floor
  Logical Operator : Logic  AllPortsSameDT=off  OutDataTypeStr=boolean
  Relational Operator : RelationalOperator  Operator=~=  OutDataTypeStr=boolean  InputSameDT=off
  Relational Operator1 : RelationalOperator  Operator===  OutDataTypeStr=boolean  InputSameDT=off
  Unit Delay : UnitDelay  SampleTime=-1  HasFrameUpgradeWarning=on
  Q : Outport
  wires:
  CLK/1 -> Data Type Conversion1/1
  Unit Delay/1 -> Relational Operator/1
  Relational Operator/1 -> Logical Operator/1
  Relational Operator1/1 -> Logical Operator/2
  Logical Operator/1 -> Q/1
  Constant/1 -> Relational Operator1/2
  Data Type Conversion1/1 -> Unit Delay/1, Relational Operator/2, Relational Operator1/1

== system Kitchen_Lib/Kitchen/100ms/Kitchn/Subsystem1/Subsystem19/Trfr/002_FlipFlop/TurnOnByButton/RisingEdgeDetection ==
  CLK : Inport
  Constant : Constant  Value=boolean(1)  OutDataTypeStr=boolean
  Data Type Conversion1 : DataTypeConversion  OutDataTypeStr=boolean  SaturateOnIntegerOverflow=off  RndMeth=Floor
  Logical Operator : Logic  AllPortsSameDT=off  OutDataTypeStr=boolean
  Relational Operator : RelationalOperator  Operator=~=  OutDataTypeStr=boolean  InputSameDT=off
  Relational Operator1 : RelationalOperator  Operator===  OutDataTypeStr=boolean  InputSameDT=off
  Unit Delay : UnitDelay  SampleTime=-1  HasFrameUpgradeWarning=on
  Q : Outport
  wires:
  CLK/1 -> Data Type Conversion1/1
  Unit Delay/1 -> Relational Operator/1
  Relational Operator/1 -> Logical Operator/1
  Relational Operator1/1 -> Logical Operator/2
  Logical Operator/1 -> Q/1
  Constant/1 -> Relational Operator1/2
  Data Type Conversion1/1 -> Unit Delay/1, Relational Operator/2, Relational Operator1/1

== system Kitchen_Lib/Kitchen/100ms/Kitchn/Subsystem1/Subsystem19/Trfr/002_FlipFlop/TurnOnNvm/RisingEdgeDetection3 ==
  CLK : Inport
  Constant : Constant  Value=boolean(1)  OutDataTypeStr=boolean
  Data Type Conversion1 : DataTypeConversion  OutDataTypeStr=boolean  SaturateOnIntegerOverflow=off  RndMeth=Floor
  Logical Operator : Logic  AllPortsSameDT=off  OutDataTypeStr=boolean
  Relational Operator : RelationalOperator  Operator=~=  OutDataTypeStr=boolean  InputSameDT=off
  Relational Operator1 : RelationalOperator  Operator===  OutDataTypeStr=boolean  InputSameDT=off
  Unit Delay : UnitDelay  SampleTime=-1  HasFrameUpgradeWarning=on
  Q : Outport
  wires:
  CLK/1 -> Data Type Conversion1/1
  Unit Delay/1 -> Relational Operator/1
  Relational Operator/1 -> Logical Operator/1
  Relational Operator1/1 -> Logical Operator/2
  Logical Operator/1 -> Q/1
  Constant/1 -> Relational Operator1/2
  Data Type Conversion1/1 -> Unit Delay/1, Relational Operator/2, Relational Operator1/1

== system Kitchen_Lib/Kitchen/100ms/Kitchn/Subsystem1/Subsystem19/Trfr/002_FlipFlop/TurnOnNvm/RisingEdgeDetection4 ==
  CLK : Inport
  Constant : Constant  Value=boolean(1)  OutDataTypeStr=boolean
  Data Type Conversion1 : DataTypeConversion  OutDataTypeStr=boolean  SaturateOnIntegerOverflow=off  RndMeth=Floor
  Logical Operator : Logic  AllPortsSameDT=off  OutDataTypeStr=boolean
  Relational Operator : RelationalOperator  Operator=~=  OutDataTypeStr=boolean  InputSameDT=off
  Relational Operator1 : RelationalOperator  Operator===  OutDataTypeStr=boolean  InputSameDT=off
  Unit Delay : UnitDelay  SampleTime=-1  HasFrameUpgradeWarning=on
  Q : Outport
  wires:
  CLK/1 -> Data Type Conversion1/1
  Unit Delay/1 -> Relational Operator/1
  Relational Operator/1 -> Logical Operator/1
  Relational Operator1/1 -> Logical Operator/2
  Logical Operator/1 -> Q/1
  Constant/1 -> Relational Operator1/2
  Data Type Conversion1/1 -> Unit Delay/1, Relational Operator/2, Relational Operator1/1
